simulink model "currloop"  (R2021b)
settings: Solver=FixedStepAuto  StartTime=0.0  StopTime=10.0  FixedStep=1e-4  RelTol=1e-3
undefined symbols (not defined in the file or in its folder): CurrKi, CurrKp, DiscIntNeverNeededParam, Pn, Ubus
libraries: slpidlib x4, mcbplantlib x1, autolibpmsmexterior x1
settings Model: DataDictionary=currloop.sldd  Creator=ssc  LastModifiedBy=ssc
settings OptimizationCC: DefaultParameterBehavior=Inlined  UseDivisionForNetSlopeComputation=on  GainParamInheritBuiltInType=on  UseFloatMulNetSlope=on  InlineInvariantSignals=on  PassReuseOutputArgsAs=Individual arguments  ZeroExternalMemoryAtStartup=off  ZeroInternalMemoryAtStartup=off  NoFixptDivByZeroProtection=on  EfficientFloat2IntCast=on  LifeSpan=1  OptimizeBlockOrder=speed  DifferentSizesBufferReuse=on  EfficientTunableParamExpr=on
settings DebuggingCC: ParameterTunabilityLossMsg=error
settings HardwareCC: ProdBitPerPointer=32  ProdBitPerSizeT=32  ProdBitPerPtrDiffT=32  ProdLargestAtomicInteger=Long  ProdLargestAtomicFloat=Double  ProdWordSize=32  ProdLongLongMode=on  ProdHWDeviceType=ARM Compatible->ARM Cortex-M
settings SFSimCC: MATLABDynamicMemAlloc=off
settings RTWCC: Description=Embedded Coder  SystemTargetFile=ert.tlc  TemplateMakefile=ert_default_tmf  GenerateReport=on  LaunchReport=on
settings CodeAppCC: ForceParamTrailComments=on  IgnoreCustomStorageClasses=off  OperatorAnnotations=on  SimulinkDataObjDesc=on  SFDataObjDesc=on  CustomSymbolStrGlobalVar=rt$N$M  CustomSymbolStrType=$N$M  CustomSymbolStrFcn=$N$M$F  CustomSymbolStrMacro=$N$M  InsertBlockDesc=on
settings ERTTargetCC: TargetLangStandard=C99 (ISO)  CodeReplacementLibrary=ARM Cortex-M  GenerateSampleERTMain=on  IncludeMdlTerminateFcn=off  CombineSignalStateStructs=on  SupportAbsoluteTime=off  SupportComplex=off  SupportContinuousTime=on  SupportNonInlinedSFcns=on  InlinedParameterPlacement=NonHierarchical  ERTCustomFileTemplate=example_file_process.tlc  ERTFilePackagingFormat=CompactWithDataFile

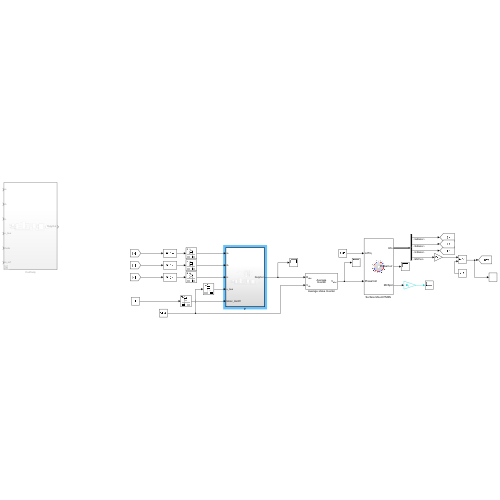
[thumbnail: Simulink's stored preview of the top-level diagram]
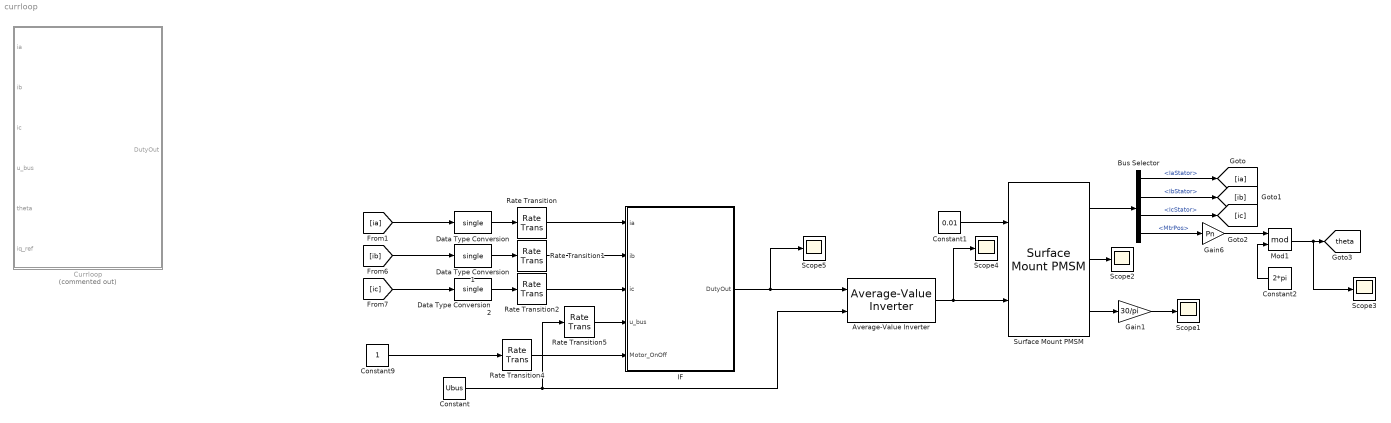
== system currloop ==
  Average-Value Inverter : mcbplantlib/Average-Value Inverter
  Bus Selector : BusSelector  OutputSignals=IaStator,IbStator,IcStator,MtrPos
  Constant : Constant  Value=Ubus
  Constant1 : Constant  Value=0.01
  Constant2 : Constant  Value=2*pi  OutDataTypeStr=single
  Constant9 : Constant
  Currloop : Subsystem  Commented=on  TreatAsAtomicUnit=on
  Data Type Conversion : DataTypeConversion  OutDataTypeStr=single
  Data Type Conversion1 : DataTypeConversion  OutDataTypeStr=single
  Data Type Conversion2 : DataTypeConversion  OutDataTypeStr=single
  Gain1 : Gain  Gain=30/pi  OutDataTypeStr=single
  Gain6 : Gain  Gain=Pn  OutDataTypeStr=single
  IF : Subsystem  TreatAsAtomicUnit=on
  Mod1 : Math  Operator=mod  OutputSignalType=real  SaturateOnIntegerOverflow=on
  Rate Transition{,1..2,4..5} (5 alike) : RateTransition
  Scope{1..5} (5 alike) : Scope
  Surface Mount PMSM : autolibpmsmexterior/Surface Mount PMSM  port_config=Torque  sim_type=Continuous  Ts=0.001  P=Pn  Rs=Rs  Ldq_=L  KConstText=Permanent flux linkage constant (lambda_pm):  lambda_pm=flux  Ke=159.9771  Kt=1.323  mechanical=[75e-6,8e-5,0]  idq0=[0 0]  theta_init=0  omega_init=0  KConst=flux  lambda_pm_calc=flux  RefBlkName='autolibpmsmexterior/Surface Mount PMSM'  aMode=5  Ldq="[0.0017      0.0017]"
      settings: SourceProductBaseCode=PW,DR,MT,UV,VE
  tag scope: theta=global
  wires:
  Average-Value Inverter/1 -> Scope4/1, Surface Mount PMSM/2
  Constant/1 -> Average-Value Inverter/2, Rate Transition5/1
  Mod1/1 -> Scope3/1, [theta]
  Bus Selector/1 -> [ia]  "<IaStator>"
  Bus Selector/4 -> Gain6/1  "<MtrPos>"
  Constant2/1 -> Mod1/2
  Surface Mount PMSM/1 -> Bus Selector/1
  Gain6/1 -> Mod1/1
  Bus Selector/3 -> [ic]  "<IcStator>"
  Bus Selector/2 -> [ib]  "<IbStator>"
  Data Type Conversion1/1 -> Rate Transition1/1
  Data Type Conversion/1 -> Rate Transition/1
  [ic] -> Data Type Conversion2/1
  [ia] -> Data Type Conversion/1
  [ib] -> Data Type Conversion1/1
  Data Type Conversion2/1 -> Rate Transition2/1
  Surface Mount PMSM/3 -> Gain1/1
  Gain1/1 -> Scope1/1
  Surface Mount PMSM/2 -> Scope2/1
  Constant9/1 -> Rate Transition4/1
  Rate Transition5/1 -> IF/4(u_bus)
  Rate Transition4/1 -> IF/5(Motor_OnOff)
  Rate Transition/1 -> IF/1(ia)
  Rate Transition1/1 -> IF/2(ib)
  Rate Transition2/1 -> IF/3(ic)
  IF/1(DutyOut) -> Scope5/1, Average-Value Inverter/1
  Constant1/1 -> Surface Mount PMSM/1

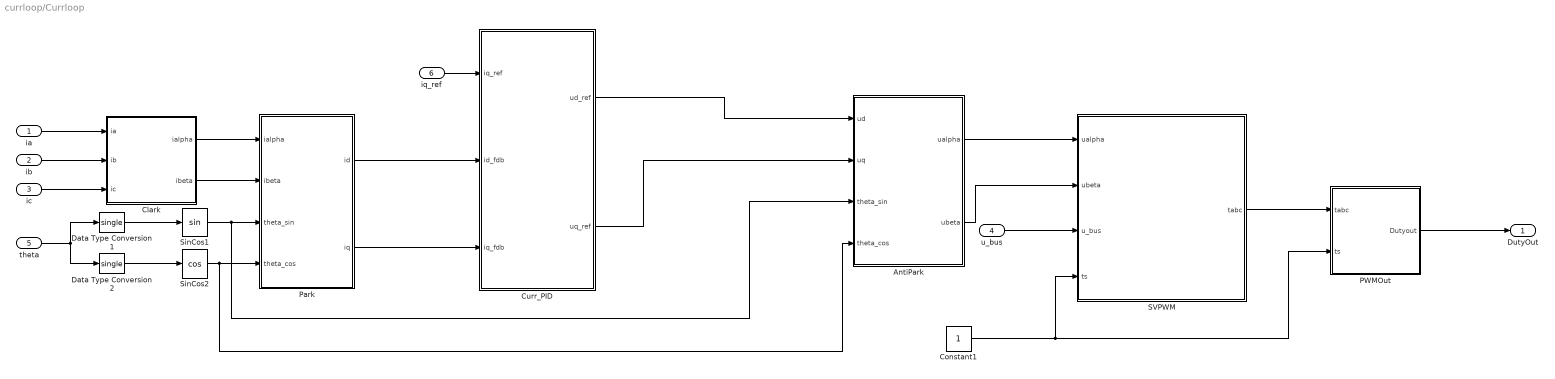
== system currloop/Currloop ==
  ia : Inport
  ib : Inport  Port=2
  ic : Inport  Port=3
  u_bus : Inport  Port=4
  theta : Inport  Port=5
  iq_ref : Inport  Port=6
  AntiPark : Subsystem
  Clark : Subsystem
  Constant1 : Constant
  Curr_PID : Subsystem
  Data Type Conversion1 : DataTypeConversion  OutDataTypeStr=single
  Data Type Conversion2 : DataTypeConversion  OutDataTypeStr=single
  PWMOut : Subsystem
  Park : Subsystem
  SVPWM : Subsystem
  SinCos1 : Trigonometry
  SinCos2 : Trigonometry  Operator=cos
  DutyOut : Outport
  wires:
  Constant1/1 -> PWMOut/2(ts), SVPWM/4(ts)
  SVPWM/1(tabc) -> PWMOut/1(tabc)
  u_bus/1 -> SVPWM/3(u_bus)
  PWMOut/1(Dutyout) -> DutyOut/1
  AntiPark/1(ualpha) -> SVPWM/1(ualpha)
  AntiPark/2(ubeta) -> SVPWM/2(ubeta)
  ia/1 -> Clark/1(ia)
  ib/1 -> Clark/2(ib)
  ic/1 -> Clark/3(ic)
  Clark/1(ialpha) -> Park/1(ialpha)
  Clark/2(ibeta) -> Park/2(ibeta)
  Park/1(id) -> Curr_PID/2(id_fdb)
  Park/2(iq) -> Curr_PID/3(iq_fdb)
  Data Type Conversion2/1 -> SinCos2/1
  Data Type Conversion1/1 -> SinCos1/1
  SinCos2/1 -> AntiPark/4(theta_cos), Park/4(theta_cos)
  SinCos1/1 -> AntiPark/3(theta_sin), Park/3(theta_sin)
  theta/1 -> Data Type Conversion1/1, Data Type Conversion2/1
  iq_ref/1 -> Curr_PID/1(iq_ref)
  Curr_PID/1(ud_ref) -> AntiPark/1(ud)
  Curr_PID/2(uq_ref) -> AntiPark/2(uq)

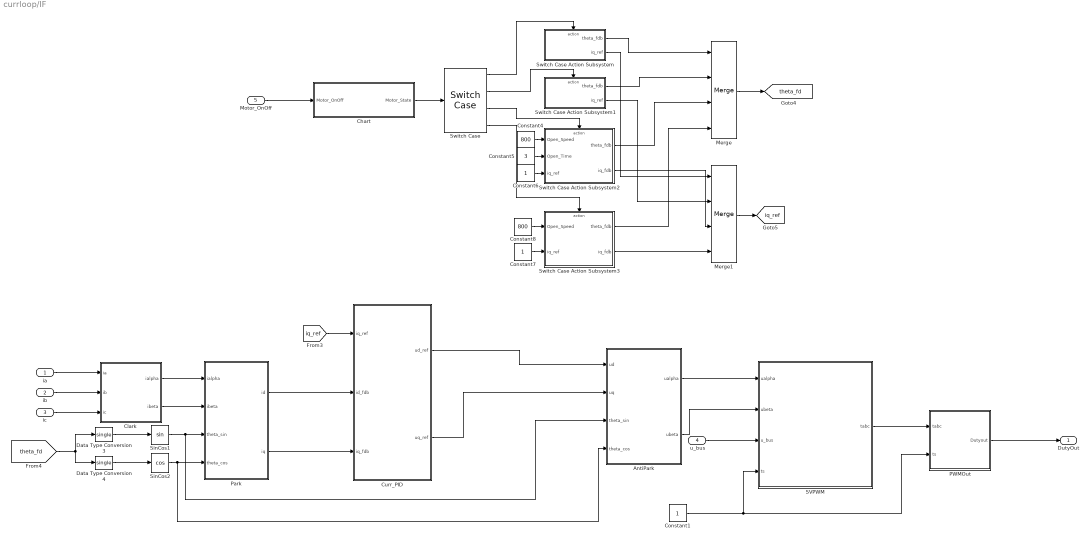
== system currloop/IF ==
  ia : Inport
  ib : Inport  Port=2
  ic : Inport  Port=3
  u_bus : Inport  Port=4
  Motor_OnOff : Inport  Port=5
  AntiPark : Subsystem
  Chart : Stateflow chart  TreatAsAtomicUnit=on
  Clark : Subsystem
  Constant1 : Constant
  Constant4 : Constant  Value=800
  Constant5 : Constant  Value=3
  Constant6 : Constant
  Constant7 : Constant
  Constant8 : Constant  Value=800
  Curr_PID : Subsystem
  Data Type Conversion3 : DataTypeConversion  OutDataTypeStr=single
  Data Type Conversion4 : DataTypeConversion  OutDataTypeStr=single
  Merge : Merge  Inputs=4
  Merge1 : Merge  Inputs=4
  PWMOut : Subsystem
  Park : Subsystem
  SVPWM : Subsystem
  SinCos1 : Trigonometry
  SinCos2 : Trigonometry  Operator=cos
  Switch Case : SwitchCase  CaseConditions={1,2,3,4}  ShowDefaultCase=off
  Switch Case Action Subsystem : Subsystem  TreatAsAtomicUnit=on
  Switch Case Action Subsystem1 : Subsystem  TreatAsAtomicUnit=on
  Switch Case Action Subsystem2 : Subsystem  TreatAsAtomicUnit=on
  Switch Case Action Subsystem3 : Subsystem  TreatAsAtomicUnit=on
  DutyOut : Outport
  tag scope: iq_ref=global, theta_fd=global
  wires:
  [iq_ref] -> Curr_PID/1(iq_ref)
  Switch Case/2 -> Switch Case Action Subsystem1/Action
  ib/1 -> Clark/2(ib)
  Park/1(id) -> Curr_PID/2(id_fdb)
  Curr_PID/1(ud_ref) -> AntiPark/1(ud)
  Clark/1(ialpha) -> Park/1(ialpha)
  Switch Case Action Subsystem/2(iq_ref) -> Merge1/1
  Data Type Conversion4/1 -> SinCos2/1
  Curr_PID/2(uq_ref) -> AntiPark/2(uq)
  [theta_fd] -> Data Type Conversion3/1, Data Type Conversion4/1
  SinCos2/1 -> AntiPark/4(theta_cos), Park/4(theta_cos)
  SinCos1/1 -> AntiPark/3(theta_sin), Park/3(theta_sin)
  AntiPark/1(ualpha) -> SVPWM/1(ualpha)
  ia/1 -> Clark/1(ia)
  Switch Case/4 -> Switch Case Action Subsystem3/Action
  Constant4/1 -> Switch Case Action Subsystem2/1(Open_Speed)
  Constant1/1 -> PWMOut/2(ts), SVPWM/4(ts)
  AntiPark/2(ubeta) -> SVPWM/2(ubeta)
  Constant8/1 -> Switch Case Action Subsystem3/1(Open_Speed)
  ic/1 -> Clark/3(ic)
  Clark/2(ibeta) -> Park/2(ibeta)
  Switch Case/3 -> Switch Case Action Subsystem2/Action
  Data Type Conversion3/1 -> SinCos1/1
  Switch Case Action Subsystem/1(theta_fdb) -> Merge/1
  SVPWM/1(tabc) -> PWMOut/1(tabc)
  Switch Case Action Subsystem1/1(theta_fdb) -> Merge/2
  Park/2(iq) -> Curr_PID/3(iq_fdb)
  u_bus/1 -> SVPWM/3(u_bus)
  Switch Case Action Subsystem3/1(theta_fdb) -> Merge/4
  Constant7/1 -> Switch Case Action Subsystem3/2(iq_ref)
  PWMOut/1(Dutyout) -> DutyOut/1
  Constant6/1 -> Switch Case Action Subsystem2/3(iq_ref)
  Switch Case/1 -> Switch Case Action Subsystem/Action
  Switch Case Action Subsystem3/2(iq_fdb) -> Merge1/4
  Merge1/1 -> [iq_ref]
  Constant5/1 -> Switch Case Action Subsystem2/2(Open_Time)
  Switch Case Action Subsystem1/2(iq_ref) -> Merge1/2
  Switch Case Action Subsystem2/1(theta_fdb) -> Merge/3
  Merge/1 -> [theta_fd]
  Switch Case Action Subsystem2/2(iq_fdb) -> Merge1/3
  Chart/1(Motor_State) -> Switch Case/1
  Motor_OnOff/1 -> Chart/1(Motor_OnOff)

== system currloop/Currloop/AntiPark ==
  ud : Inport
  uq : Inport  Port=2
  theta_sin : Inport  Port=3
  theta_cos : Inport  Port=4
  Product{,1..3} (4 alike) : Product
  Subtract : Sum
  Subtract1 : Sum  Inputs=-+
  ualpha : Outport
  ubeta : Outport  Port=2
  wires:
  ud/1 -> Product/1, Product3/1
  theta_sin/1 -> Product2/2, Product/2
  uq/1 -> Product1/1, Product2/1
  theta_cos/1 -> Product3/2, Product1/2
  Product/1 -> Subtract/1
  Product1/1 -> Subtract/2
  Product2/1 -> Subtract1/1
  Product3/1 -> Subtract1/2
  Subtract/1 -> ubeta/1
  Subtract1/1 -> ualpha/1

== system currloop/Currloop/Clark ==
  ia : Inport
  ib : Inport  Port=2
  ic : Inport  Port=3
  Add : Sum
  Add1 : Sum  Inputs=+-
  Add2 : Sum  Inputs=+-
  Gain : Gain  Gain=2/3
  Gain1 : Gain  Gain=1/3
  Gain2 : Gain  Gain=sqrt(3)/3
  ialpha : Outport
  ibeta : Outport  Port=2
  wires:
  ia/1 -> Gain/1
  ib/1 -> Add1/1, Add/1
  ic/1 -> Add1/2, Add/2
  Add/1 -> Gain1/1
  Add1/1 -> Gain2/1
  Gain1/1 -> Add2/2
  Gain/1 -> Add2/1
  Gain2/1 -> ibeta/1
  Add2/1 -> ialpha/1

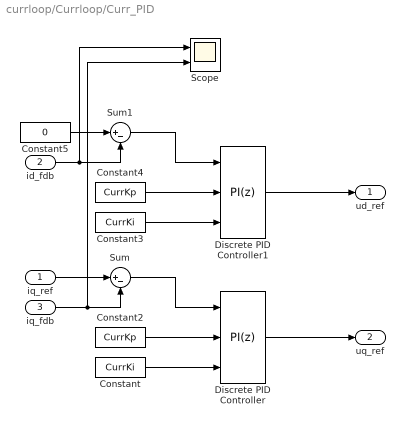
== system currloop/Currloop/Curr_PID ==
  iq_ref : Inport
  id_fdb : Inport  Port=2
  iq_fdb : Inport  Port=3
  Constant : Constant  Value=CurrKi
  Constant2 : Constant  Value=CurrKp
  Constant3 : Constant  Value=CurrKi
  Constant4 : Constant  Value=CurrKp
  Constant5 : Constant  Value=0
  Discrete PID Controller : slpidlib/PID Controller  Controller=PI  Form=Parallel  TimeDomain=Discrete-time  UseExternalTs=off  SampleTime=-1  IntegratorMethod=Forward Euler  FilterMethod=Forward Euler  ControllerParametersSource=external  P=1  I=1  D=0  UseFilter=on  N=100  TunerSelectOption=Transfer Function Based (PID Tuner App)  InitialConditionSource=internal  InitialConditionForIntegrator=0  InitialConditionForFilter=0  DifferentiatorICPrevScaledInput=0  ExternalReset=none  TrackingMode=off  Kt=1  LimitOutput=on  SatLimitsSource=internal  UpperSaturationLimit=Ubus/sqrt(3)  LowerSaturationLimit=-Ubus/sqrt(3)  LinearizeAsGain=off  AntiWindupMode=clamping  Kb=1  POutMin=[]  POutMax=[]  IOutMin=[]  IOutMax=[]  DOutMin=[]  DOutMax=[]  NOutMin=[]  NOutMax=[]  SumOutMin=[]  SumOutMax=[]  SaturationOutMin=[]  SaturationOutMax=[]  PParamMin=[]  PParamMax=[]  IParamMin=[]  IParamMax=[]  DParamMin=[]  DParamMax=[]  NParamMin=[]  NParamMax=[]  KbParamMin=[]  KbParamMax=[]  KtParamMin=[]  KtParamMax=[]  KbOutMin=[]  KbOutMax=[]  KtOutMin=[]  KtOutMax=[]  IntegratorOutMin=[]  IntegratorOutMax=[]  FilterOutMin=[]  FilterOutMax=[]  SumI1OutMin=[]  SumI1OutMax=[]  SumI2OutMin=[]  SumI2OutMax=[]  SumI3OutMin=[]  SumI3OutMax=[]  SumI4OutMin=[]  SumI4OutMax=[]  SumDOutMin=[]  SumDOutMax=[]  DifferentiatorOutMin=[]  DifferentiatorOutMax=[]  FilterDiffOutCoefMin=[]  FilterDiffOutCoefMax=[]  ReciprocalOutMin=[]  ReciprocalOutMax=[]  SumDenOutMin=[]  SumDenOutMax=[]  SumNumOutMin=[]  SumNumOutMax=[]  DivideOutMin=[]  DivideOutMax=[]  UdiffTsProdOutMin=[]  UdiffTsProdOutMax=[]  NTsProdOutMin=[]  NTsProdOutMax=[]  UintegralTsProdOutMin=[]  UintegralTsProdOutMax=[]  UngainTsProdOutMin=[]  UngainTsProdOutMax=[]  IntegratorContinuousStateAttributes=''  IntegratorStateMustResolveToSignalObject=off  IntegratorRTWStateStorageClass=Auto  FilterContinuousStateAttributes=''  FilterStateMustResolveToSignalObject=off  FilterRTWStateStorageClass=Auto  ParallelPVariant=ExternalParameters  IdealPVariant=Disabled  IVariant=ExternalParameters  DVariant=Disabled  IntegratorVariant=Discrete  SatVariant=Enabled  AWVariant=DiscClampingParallel  PCopyVariant=Disabled  TRVariant=Disabled  FdbkBlocksVariant=Forward  IdealPFdbkVariant=Disabled  SatFdbkVariant=Disabled  DerivativeFilterVariant=Disabled  NVariant=Disabled  NCopyVariant=Disabled_SignalSpec  FilterICVariant=Disabled  IntegratorICVariant=InternalICs  ExternalResetVariant=Disabled  TRSumVariant=Passthrough  SumFdbkVariant=Disabled  SumVariant=Sum_PI  TsampFilterVariant=InternalTs  TsampNgainVariant=Passthrough  TsampIntegralVariant=Passthrough  ExternalSaturationOutDataTypeStr=Inherit: Same as second input
  Discrete PID Controller1 : slpidlib/PID Controller  Controller=PI  Form=Parallel  TimeDomain=Discrete-time  UseExternalTs=off  SampleTime=-1  IntegratorMethod=Forward Euler  FilterMethod=Forward Euler  ControllerParametersSource=external  P=1  I=1  D=0  UseFilter=on  N=100  TunerSelectOption=Transfer Function Based (PID Tuner App)  InitialConditionSource=internal  InitialConditionForIntegrator=0  InitialConditionForFilter=0  DifferentiatorICPrevScaledInput=0  ExternalReset=none  TrackingMode=off  Kt=1  LimitOutput=on  SatLimitsSource=internal  UpperSaturationLimit=Ubus/sqrt(3)  LowerSaturationLimit=-Ubus/sqrt(3)  LinearizeAsGain=off  AntiWindupMode=clamping  Kb=1  POutMin=[]  POutMax=[]  IOutMin=[]  IOutMax=[]  DOutMin=[]  DOutMax=[]  NOutMin=[]  NOutMax=[]  SumOutMin=[]  SumOutMax=[]  SaturationOutMin=[]  SaturationOutMax=[]  PParamMin=[]  PParamMax=[]  IParamMin=[]  IParamMax=[]  DParamMin=[]  DParamMax=[]  NParamMin=[]  NParamMax=[]  KbParamMin=[]  KbParamMax=[]  KtParamMin=[]  KtParamMax=[]  KbOutMin=[]  KbOutMax=[]  KtOutMin=[]  KtOutMax=[]  IntegratorOutMin=[]  IntegratorOutMax=[]  FilterOutMin=[]  FilterOutMax=[]  SumI1OutMin=[]  SumI1OutMax=[]  SumI2OutMin=[]  SumI2OutMax=[]  SumI3OutMin=[]  SumI3OutMax=[]  SumI4OutMin=[]  SumI4OutMax=[]  SumDOutMin=[]  SumDOutMax=[]  DifferentiatorOutMin=[]  DifferentiatorOutMax=[]  FilterDiffOutCoefMin=[]  FilterDiffOutCoefMax=[]  ReciprocalOutMin=[]  ReciprocalOutMax=[]  SumDenOutMin=[]  SumDenOutMax=[]  SumNumOutMin=[]  SumNumOutMax=[]  DivideOutMin=[]  DivideOutMax=[]  UdiffTsProdOutMin=[]  UdiffTsProdOutMax=[]  NTsProdOutMin=[]  NTsProdOutMax=[]  UintegralTsProdOutMin=[]  UintegralTsProdOutMax=[]  UngainTsProdOutMin=[]  UngainTsProdOutMax=[]  IntegratorContinuousStateAttributes=''  IntegratorStateMustResolveToSignalObject=off  IntegratorRTWStateStorageClass=Auto  FilterContinuousStateAttributes=''  FilterStateMustResolveToSignalObject=off  FilterRTWStateStorageClass=Auto  ParallelPVariant=ExternalParameters  IdealPVariant=Disabled  IVariant=ExternalParameters  DVariant=Disabled  IntegratorVariant=Discrete  SatVariant=Enabled  AWVariant=DiscClampingParallel  PCopyVariant=Disabled  TRVariant=Disabled  FdbkBlocksVariant=Forward  IdealPFdbkVariant=Disabled  SatFdbkVariant=Disabled  DerivativeFilterVariant=Disabled  NVariant=Disabled  NCopyVariant=Disabled_SignalSpec  FilterICVariant=Disabled  IntegratorICVariant=InternalICs  ExternalResetVariant=Disabled  TRSumVariant=Passthrough  SumFdbkVariant=Disabled  SumVariant=Sum_PI  TsampFilterVariant=InternalTs  TsampNgainVariant=Passthrough  TsampIntegralVariant=Passthrough  ExternalSaturationOutDataTypeStr=Inherit: Same as second input
  Scope : Scope  NumInputPorts=2
  Sum : Sum  Inputs=|+-
  Sum1 : Sum  Inputs=|+-
  ud_ref : Outport
  uq_ref : Outport  Port=2
  wires:
  Constant2/1 -> Discrete PID Controller/2
  Constant3/1 -> Discrete PID Controller1/3
  Sum1/1 -> Discrete PID Controller1/1
  Sum/1 -> Discrete PID Controller/1
  Constant/1 -> Discrete PID Controller/3
  iq_ref/1 -> Sum/1
  Discrete PID Controller/1 -> uq_ref/1
  Constant4/1 -> Discrete PID Controller1/2
  Discrete PID Controller1/1 -> ud_ref/1
  Constant5/1 -> Sum1/1
  iq_fdb/1 -> Scope/2, Sum/2
  id_fdb/1 -> Scope/1, Sum1/2

== system currloop/Currloop/PWMOut ==
  tabc : Inport
  ts : Inport  Port=2
  Add : Sum  Inputs=-+
  Add1 : Sum  Inputs=-+
  Add2 : Sum  Inputs=-+
  Demux : Demux  Outputs=3
  Divide : Product  Inputs=*/
  Divide1 : Product  Inputs=*/
  Divide2 : Product  Inputs=*/
  Gain : Gain  Gain=2
  Mux : Mux  Inputs=3
  Dutyout : Outport
  wires:
  tabc/1 -> Gain/1
  Gain/1 -> Demux/1
  ts/1 -> Add1/2, Add2/2, Add/2, Divide2/2, Divide1/2, Divide/2
  Demux/3 -> Add/1
  Add/1 -> Divide/1
  Divide/1 -> Mux/3  "Dutyc"
  Demux/1 -> Add2/1
  Add1/1 -> Divide1/1
  Add2/1 -> Divide2/1
  Demux/2 -> Add1/1
  Divide1/1 -> Mux/2  "Dutyb"
  Divide2/1 -> Mux/1  "Dutya"
  Mux/1 -> Dutyout/1

== system currloop/Currloop/Park ==
  ialpha : Inport
  ibeta : Inport  Port=2
  theta_sin : Inport  Port=3
  theta_cos : Inport  Port=4
  Product{,1..3} (4 alike) : Product
  Subtract : Sum
  Subtract1 : Sum  Inputs=-+
  id : Outport
  iq : Outport  Port=2
  wires:
  ialpha/1 -> Product2/1, Product/1
  theta_cos/1 -> Product/2, Product3/2
  ibeta/1 -> Product3/1, Product1/1
  theta_sin/1 -> Product1/2, Product2/2
  Product/1 -> Subtract/1
  Product1/1 -> Subtract/2
  Subtract/1 -> id/1
  Product2/1 -> Subtract1/1
  Product3/1 -> Subtract1/2
  Subtract1/1 -> iq/1

== system currloop/Currloop/SVPWM ==
  ualpha : Inport
  ubeta : Inport  Port=2
  u_bus : Inport  Port=3
  ts : Inport  Port=4
  N : Subsystem
  t4_t6 : Subsystem
  t_abc : Subsystem
  tabc : Outport
  wires:
  ubeta/1 -> t4_t6/2(ubeta), N/2(ubeta)
  t4_t6/1(t4) -> t_abc/1(t4)
  N/1(N) -> t_abc/4(N), t4_t6/4(N)
  ualpha/1 -> t4_t6/1(ualpha), N/1(ualpha)
  t4_t6/2(t6) -> t_abc/2(t6)
  u_bus/1 -> t4_t6/3(u_bus)
  ts/1 -> t_abc/3(ts), t4_t6/5(ts)
  t_abc/1(tabc) -> tabc/1

== system currloop/IF/AntiPark ==
  ud : Inport
  uq : Inport  Port=2
  theta_sin : Inport  Port=3
  theta_cos : Inport  Port=4
  Product{,1..3} (4 alike) : Product
  Subtract : Sum
  Subtract1 : Sum  Inputs=-+
  ualpha : Outport
  ubeta : Outport  Port=2
  wires:
  ud/1 -> Product/1, Product3/1
  theta_sin/1 -> Product2/2, Product/2
  uq/1 -> Product1/1, Product2/1
  theta_cos/1 -> Product3/2, Product1/2
  Product/1 -> Subtract/1
  Product1/1 -> Subtract/2
  Product2/1 -> Subtract1/1
  Product3/1 -> Subtract1/2
  Subtract/1 -> ubeta/1
  Subtract1/1 -> ualpha/1

== system currloop/IF/Clark ==
  ia : Inport
  ib : Inport  Port=2
  ic : Inport  Port=3
  Add : Sum
  Add1 : Sum  Inputs=+-
  Add2 : Sum  Inputs=+-
  Gain : Gain  Gain=2/3
  Gain1 : Gain  Gain=1/3
  Gain2 : Gain  Gain=sqrt(3)/3
  ialpha : Outport
  ibeta : Outport  Port=2
  wires:
  ia/1 -> Gain/1
  ib/1 -> Add1/1, Add/1
  ic/1 -> Add1/2, Add/2
  Add/1 -> Gain1/1
  Add1/1 -> Gain2/1
  Gain1/1 -> Add2/2
  Gain/1 -> Add2/1
  Gain2/1 -> ibeta/1
  Add2/1 -> ialpha/1

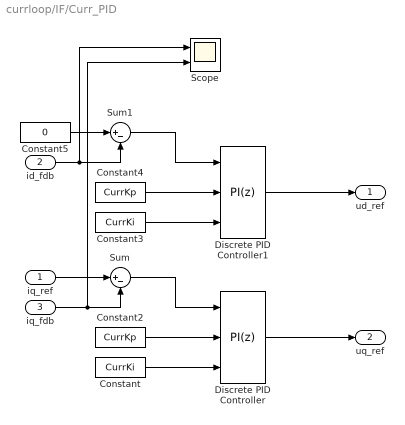
== system currloop/IF/Curr_PID ==
  iq_ref : Inport
  id_fdb : Inport  Port=2
  iq_fdb : Inport  Port=3
  Constant : Constant  Value=CurrKi
  Constant2 : Constant  Value=CurrKp
  Constant3 : Constant  Value=CurrKi
  Constant4 : Constant  Value=CurrKp
  Constant5 : Constant  Value=0
  Discrete PID Controller : slpidlib/PID Controller  Controller=PI  Form=Parallel  TimeDomain=Discrete-time  UseExternalTs=off  SampleTime=-1  IntegratorMethod=Forward Euler  FilterMethod=Forward Euler  ControllerParametersSource=external  P=1  I=1  D=0  UseFilter=on  N=100  TunerSelectOption=Transfer Function Based (PID Tuner App)  InitialConditionSource=internal  InitialConditionForIntegrator=0  InitialConditionForFilter=0  DifferentiatorICPrevScaledInput=0  ExternalReset=none  TrackingMode=off  Kt=1  LimitOutput=on  SatLimitsSource=internal  UpperSaturationLimit=Ubus/sqrt(3)  LowerSaturationLimit=-Ubus/sqrt(3)  LinearizeAsGain=off  AntiWindupMode=clamping  Kb=1  POutMin=[]  POutMax=[]  IOutMin=[]  IOutMax=[]  DOutMin=[]  DOutMax=[]  NOutMin=[]  NOutMax=[]  SumOutMin=[]  SumOutMax=[]  SaturationOutMin=[]  SaturationOutMax=[]  PParamMin=[]  PParamMax=[]  IParamMin=[]  IParamMax=[]  DParamMin=[]  DParamMax=[]  NParamMin=[]  NParamMax=[]  KbParamMin=[]  KbParamMax=[]  KtParamMin=[]  KtParamMax=[]  KbOutMin=[]  KbOutMax=[]  KtOutMin=[]  KtOutMax=[]  IntegratorOutMin=[]  IntegratorOutMax=[]  FilterOutMin=[]  FilterOutMax=[]  SumI1OutMin=[]  SumI1OutMax=[]  SumI2OutMin=[]  SumI2OutMax=[]  SumI3OutMin=[]  SumI3OutMax=[]  SumI4OutMin=[]  SumI4OutMax=[]  SumDOutMin=[]  SumDOutMax=[]  DifferentiatorOutMin=[]  DifferentiatorOutMax=[]  FilterDiffOutCoefMin=[]  FilterDiffOutCoefMax=[]  ReciprocalOutMin=[]  ReciprocalOutMax=[]  SumDenOutMin=[]  SumDenOutMax=[]  SumNumOutMin=[]  SumNumOutMax=[]  DivideOutMin=[]  DivideOutMax=[]  UdiffTsProdOutMin=[]  UdiffTsProdOutMax=[]  NTsProdOutMin=[]  NTsProdOutMax=[]  UintegralTsProdOutMin=[]  UintegralTsProdOutMax=[]  UngainTsProdOutMin=[]  UngainTsProdOutMax=[]  IntegratorContinuousStateAttributes=''  IntegratorStateMustResolveToSignalObject=off  IntegratorRTWStateStorageClass=Auto  FilterContinuousStateAttributes=''  FilterStateMustResolveToSignalObject=off  FilterRTWStateStorageClass=Auto  ParallelPVariant=ExternalParameters  IdealPVariant=Disabled  IVariant=ExternalParameters  DVariant=Disabled  IntegratorVariant=Discrete  SatVariant=Enabled  AWVariant=DiscClampingParallel  PCopyVariant=Disabled  TRVariant=Disabled  FdbkBlocksVariant=Forward  IdealPFdbkVariant=Disabled  SatFdbkVariant=Disabled  DerivativeFilterVariant=Disabled  NVariant=Disabled  NCopyVariant=Disabled_SignalSpec  FilterICVariant=Disabled  IntegratorICVariant=InternalICs  ExternalResetVariant=Disabled  TRSumVariant=Passthrough  SumFdbkVariant=Disabled  SumVariant=Sum_PI  TsampFilterVariant=InternalTs  TsampNgainVariant=Passthrough  TsampIntegralVariant=Passthrough  ExternalSaturationOutDataTypeStr=Inherit: Same as second input
  Discrete PID Controller1 : slpidlib/PID Controller  Controller=PI  Form=Parallel  TimeDomain=Discrete-time  UseExternalTs=off  SampleTime=-1  IntegratorMethod=Forward Euler  FilterMethod=Forward Euler  ControllerParametersSource=external  P=1  I=1  D=0  UseFilter=on  N=100  TunerSelectOption=Transfer Function Based (PID Tuner App)  InitialConditionSource=internal  InitialConditionForIntegrator=0  InitialConditionForFilter=0  DifferentiatorICPrevScaledInput=0  ExternalReset=none  TrackingMode=off  Kt=1  LimitOutput=on  SatLimitsSource=internal  UpperSaturationLimit=Ubus/sqrt(3)  LowerSaturationLimit=-Ubus/sqrt(3)  LinearizeAsGain=off  AntiWindupMode=clamping  Kb=1  POutMin=[]  POutMax=[]  IOutMin=[]  IOutMax=[]  DOutMin=[]  DOutMax=[]  NOutMin=[]  NOutMax=[]  SumOutMin=[]  SumOutMax=[]  SaturationOutMin=[]  SaturationOutMax=[]  PParamMin=[]  PParamMax=[]  IParamMin=[]  IParamMax=[]  DParamMin=[]  DParamMax=[]  NParamMin=[]  NParamMax=[]  KbParamMin=[]  KbParamMax=[]  KtParamMin=[]  KtParamMax=[]  KbOutMin=[]  KbOutMax=[]  KtOutMin=[]  KtOutMax=[]  IntegratorOutMin=[]  IntegratorOutMax=[]  FilterOutMin=[]  FilterOutMax=[]  SumI1OutMin=[]  SumI1OutMax=[]  SumI2OutMin=[]  SumI2OutMax=[]  SumI3OutMin=[]  SumI3OutMax=[]  SumI4OutMin=[]  SumI4OutMax=[]  SumDOutMin=[]  SumDOutMax=[]  DifferentiatorOutMin=[]  DifferentiatorOutMax=[]  FilterDiffOutCoefMin=[]  FilterDiffOutCoefMax=[]  ReciprocalOutMin=[]  ReciprocalOutMax=[]  SumDenOutMin=[]  SumDenOutMax=[]  SumNumOutMin=[]  SumNumOutMax=[]  DivideOutMin=[]  DivideOutMax=[]  UdiffTsProdOutMin=[]  UdiffTsProdOutMax=[]  NTsProdOutMin=[]  NTsProdOutMax=[]  UintegralTsProdOutMin=[]  UintegralTsProdOutMax=[]  UngainTsProdOutMin=[]  UngainTsProdOutMax=[]  IntegratorContinuousStateAttributes=''  IntegratorStateMustResolveToSignalObject=off  IntegratorRTWStateStorageClass=Auto  FilterContinuousStateAttributes=''  FilterStateMustResolveToSignalObject=off  FilterRTWStateStorageClass=Auto  ParallelPVariant=ExternalParameters  IdealPVariant=Disabled  IVariant=ExternalParameters  DVariant=Disabled  IntegratorVariant=Discrete  SatVariant=Enabled  AWVariant=DiscClampingParallel  PCopyVariant=Disabled  TRVariant=Disabled  FdbkBlocksVariant=Forward  IdealPFdbkVariant=Disabled  SatFdbkVariant=Disabled  DerivativeFilterVariant=Disabled  NVariant=Disabled  NCopyVariant=Disabled_SignalSpec  FilterICVariant=Disabled  IntegratorICVariant=InternalICs  ExternalResetVariant=Disabled  TRSumVariant=Passthrough  SumFdbkVariant=Disabled  SumVariant=Sum_PI  TsampFilterVariant=InternalTs  TsampNgainVariant=Passthrough  TsampIntegralVariant=Passthrough  ExternalSaturationOutDataTypeStr=Inherit: Same as second input
  Scope : Scope  NumInputPorts=2
  Sum : Sum  Inputs=|+-
  Sum1 : Sum  Inputs=|+-
  ud_ref : Outport
  uq_ref : Outport  Port=2
  wires:
  Constant2/1 -> Discrete PID Controller/2
  Constant3/1 -> Discrete PID Controller1/3
  Sum1/1 -> Discrete PID Controller1/1
  Sum/1 -> Discrete PID Controller/1
  Constant/1 -> Discrete PID Controller/3
  iq_ref/1 -> Sum/1
  Discrete PID Controller/1 -> uq_ref/1
  Constant4/1 -> Discrete PID Controller1/2
  Discrete PID Controller1/1 -> ud_ref/1
  Constant5/1 -> Sum1/1
  iq_fdb/1 -> Scope/2, Sum/2
  id_fdb/1 -> Scope/1, Sum1/2

== system currloop/IF/PWMOut ==
  tabc : Inport
  ts : Inport  Port=2
  Add : Sum  Inputs=-+
  Add1 : Sum  Inputs=-+
  Add2 : Sum  Inputs=-+
  Demux : Demux  Outputs=3
  Divide : Product  Inputs=*/
  Divide1 : Product  Inputs=*/
  Divide2 : Product  Inputs=*/
  Gain : Gain  Gain=2
  Mux : Mux  Inputs=3
  Dutyout : Outport
  wires:
  tabc/1 -> Gain/1
  Gain/1 -> Demux/1
  ts/1 -> Add1/2, Add2/2, Add/2, Divide2/2, Divide1/2, Divide/2
  Demux/3 -> Add/1
  Add/1 -> Divide/1
  Divide/1 -> Mux/3  "Dutyc"
  Demux/1 -> Add2/1
  Add1/1 -> Divide1/1
  Add2/1 -> Divide2/1
  Demux/2 -> Add1/1
  Divide1/1 -> Mux/2  "Dutyb"
  Divide2/1 -> Mux/1  "Dutya"
  Mux/1 -> Dutyout/1

== system currloop/IF/Park ==
  ialpha : Inport
  ibeta : Inport  Port=2
  theta_sin : Inport  Port=3
  theta_cos : Inport  Port=4
  Product{,1..3} (4 alike) : Product
  Subtract : Sum
  Subtract1 : Sum  Inputs=-+
  id : Outport
  iq : Outport  Port=2
  wires:
  ialpha/1 -> Product2/1, Product/1
  theta_cos/1 -> Product/2, Product3/2
  ibeta/1 -> Product3/1, Product1/1
  theta_sin/1 -> Product1/2, Product2/2
  Product/1 -> Subtract/1
  Product1/1 -> Subtract/2
  Subtract/1 -> id/1
  Product2/1 -> Subtract1/1
  Product3/1 -> Subtract1/2
  Subtract1/1 -> iq/1

== system currloop/IF/SVPWM ==
  ualpha : Inport
  ubeta : Inport  Port=2
  u_bus : Inport  Port=3
  ts : Inport  Port=4
  N : Subsystem
  t4_t6 : Subsystem
  t_abc : Subsystem
  tabc : Outport
  wires:
  ubeta/1 -> t4_t6/2(ubeta), N/2(ubeta)
  t4_t6/1(t4) -> t_abc/1(t4)
  N/1(N) -> t_abc/4(N), t4_t6/4(N)
  ualpha/1 -> t4_t6/1(ualpha), N/1(ualpha)
  t4_t6/2(t6) -> t_abc/2(t6)
  u_bus/1 -> t4_t6/3(u_bus)
  ts/1 -> t_abc/3(ts), t4_t6/5(ts)
  t_abc/1(tabc) -> tabc/1

== system currloop/IF/Switch Case Action Subsystem ==
  Action Port : ActionPort  ActionPortLabel=case [ 1 ]:
  Constant : Constant  Value=0
  Constant1 : Constant  Value=0
  theta_fdb : Outport
  iq_ref : Outport  Port=2
  wires:
  Constant/1 -> theta_fdb/1
  Constant1/1 -> iq_ref/1

== system currloop/IF/Switch Case Action Subsystem1 ==
  Action Port : ActionPort  ActionPortLabel=case [ 2 ]:
  Constant : Constant  Value=0
  Constant1 : Constant
  theta_fdb : Outport
  iq_ref : Outport  Port=2
  wires:
  Constant/1 -> theta_fdb/1
  Constant1/1 -> iq_ref/1

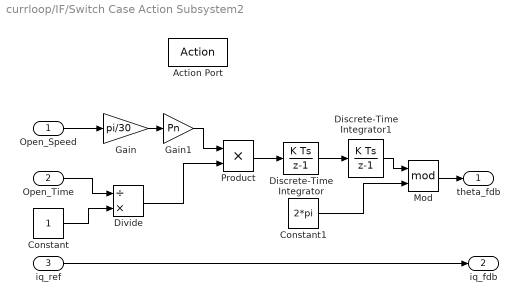
== system currloop/IF/Switch Case Action Subsystem2 ==
  Open_Speed : Inport
  Open_Time : Inport  Port=2
  iq_ref : Inport  Port=3
  Action Port : ActionPort  ActionPortLabel=case [ 3 ]:
  Constant : Constant
  Constant1 : Constant  Value=2*pi  OutDataTypeStr=double
  Discrete-Time Integrator : DiscreteIntegrator  SampleTime=-1  ICPrevOutput=DiscIntNeverNeededParam  ICPrevScaledInput=DiscIntNeverNeededParam
  Discrete-Time Integrator1 : DiscreteIntegrator  SampleTime=-1  ICPrevOutput=DiscIntNeverNeededParam  ICPrevScaledInput=DiscIntNeverNeededParam
  Divide : Product  Inputs=/*
  Gain : Gain  Gain=pi/30
  Gain1 : Gain  Gain=Pn
  Mod : Math  Operator=mod  SaturateOnIntegerOverflow=on
  Product : Product
  theta_fdb : Outport
  iq_fdb : Outport  Port=2
  wires:
  Open_Speed/1 -> Gain/1
  Gain/1 -> Gain1/1
  Gain1/1 -> Product/1
  Open_Time/1 -> Divide/1
  Constant/1 -> Divide/2
  Divide/1 -> Product/2
  Product/1 -> Discrete-Time Integrator/1
  iq_ref/1 -> iq_fdb/1
  Discrete-Time Integrator/1 -> Discrete-Time Integrator1/1
  Mod/1 -> theta_fdb/1
  Constant1/1 -> Mod/2
  Discrete-Time Integrator1/1 -> Mod/1

== system currloop/IF/Switch Case Action Subsystem3 ==
  Open_Speed : Inport
  iq_ref : Inport  Port=2
  Action Port : ActionPort  ActionPortLabel=case [ 4 ]:
  Constant1 : Constant  Value=2*pi  OutDataTypeStr=double
  Discrete-Time Integrator1 : DiscreteIntegrator  SampleTime=-1  ICPrevOutput=DiscIntNeverNeededParam  ICPrevScaledInput=DiscIntNeverNeededParam
  Gain : Gain  Gain=pi/30
  Gain1 : Gain  Gain=Pn
  Mod : Math  Operator=mod  SaturateOnIntegerOverflow=on
  theta_fdb : Outport
  iq_fdb : Outport  Port=2
  wires:
  Open_Speed/1 -> Gain/1
  Gain/1 -> Gain1/1
  iq_ref/1 -> iq_fdb/1
  Gain1/1 -> Discrete-Time Integrator1/1
  Constant1/1 -> Mod/2
  Discrete-Time Integrator1/1 -> Mod/1
  Mod/1 -> theta_fdb/1

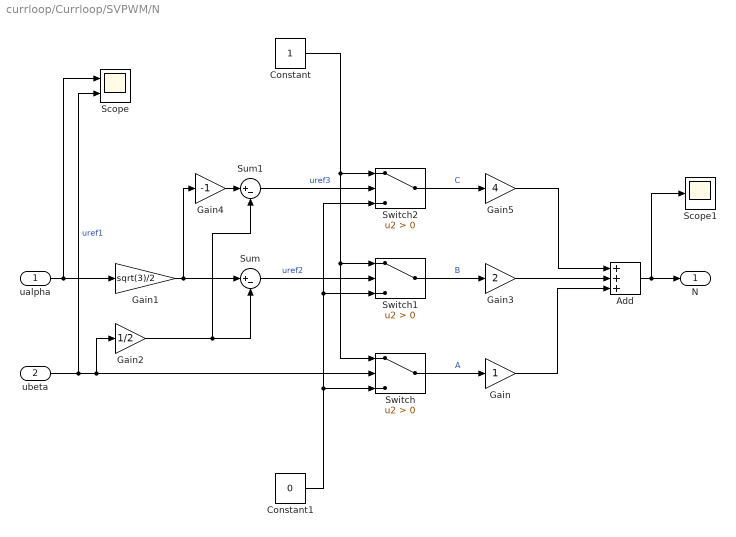
== system currloop/Currloop/SVPWM/N ==
  ualpha : Inport
  ubeta : Inport  Port=2
  Add : Sum  Inputs=+++
  Constant : Constant  OutDataTypeStr=single
  Constant1 : Constant  Value=0  OutDataTypeStr=single
  Gain : Gain
  Gain1 : Gain  Gain=sqrt(3)/2
  Gain2 : Gain  Gain=1/2
  Gain3 : Gain  Gain=2
  Gain4 : Gain  Gain=-1
  Gain5 : Gain  Gain=4
  Scope : Scope  NumInputPorts=2
  Scope1 : Scope
  Sum : Sum  Inputs=|+-
  Sum1 : Sum  Inputs=|+-
  Switch : Switch  Criteria=u2 > Threshold
  Switch1 : Switch  Criteria=u2 > Threshold
  Switch2 : Switch  Criteria=u2 > Threshold
  N : Outport
  wires:
  ualpha/1 -> Gain1/1, Scope/1
  ubeta/1 -> Switch/2, Gain2/1, Scope/2  "uref1"
  Constant/1 -> Switch2/1, Switch1/1, Switch/1
  Constant1/1 -> Switch2/3, Switch1/3, Switch/3
  Switch/1 -> Gain/1  "A"
  Gain1/1 -> Gain4/1, Sum/1
  Gain2/1 -> Sum1/2, Sum/2
  Sum/1 -> Switch1/2  "uref2"
  Switch1/1 -> Gain3/1  "B"
  Gain4/1 -> Sum1/1
  Sum1/1 -> Switch2/2  "uref3"
  Switch2/1 -> Gain5/1  "C"
  Gain3/1 -> Add/2
  Add/1 -> Scope1/1, N/1
  Gain/1 -> Add/3
  Gain5/1 -> Add/1

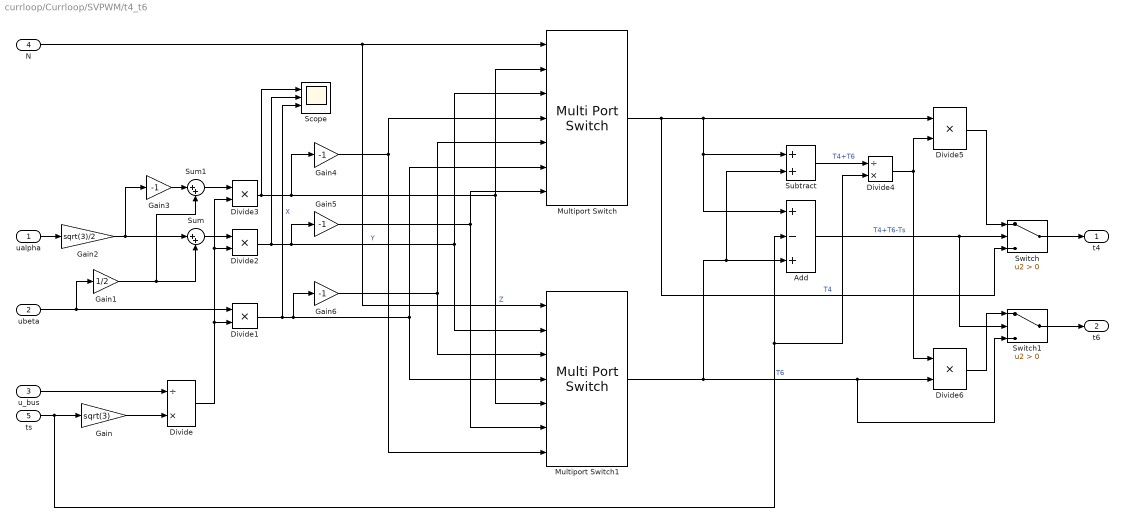
== system currloop/Currloop/SVPWM/t4_t6 ==
  ualpha : Inport
  ubeta : Inport  Port=2
  u_bus : Inport  Port=3
  N : Inport  Port=4
  ts : Inport  Port=5
  Add : Sum  Inputs=+-+
  Divide : Product  Inputs=/*
  Divide{1..3,5..6} (5 alike) : Product  Inputs=**
  Divide4 : Product  Inputs=/*
  Gain : Gain  Gain=sqrt(3)
  Gain1 : Gain  Gain=1/2
  Gain2 : Gain  Gain=sqrt(3)/2
  Gain{3..6} (4 alike) : Gain  Gain=-1
  Multiport Switch : MultiPortSwitch  Inputs=6
  Multiport Switch1 : MultiPortSwitch  Inputs=6
  Scope : Scope  NumInputPorts=3
  Subtract : Sum
  Sum : Sum  Inputs=|++
  Sum1 : Sum  Inputs=|++
  Switch : Switch  Criteria=u2 > Threshold
  Switch1 : Switch  Criteria=u2 > Threshold
  t4 : Outport
  t6 : Outport  Port=2
  wires:
  ts/1 -> Gain/1, Divide4/2, Add/2
  u_bus/1 -> Divide/1
  Gain/1 -> Divide/2
  ubeta/1 -> Gain1/1, Divide1/1
  Divide/1 -> Divide3/2, Divide2/2, Divide1/2
  Divide1/1 -> Scope/3, Multiport Switch1/4, Multiport Switch/6, Gain6/1  "X"
  ualpha/1 -> Gain2/1
  Gain1/1 -> Sum1/2, Sum/2
  Gain2/1 -> Gain3/1, Sum/1
  Sum/1 -> Divide2/1
  Divide2/1 -> Scope/2, Multiport Switch1/2, Multiport Switch/3, Gain5/1  "Y"
  Gain3/1 -> Sum1/1
  Sum1/1 -> Divide3/1
  Divide3/1 -> Scope/1, Gain4/1, Multiport Switch1/5, Multiport Switch/2  "Z"
  N/1 -> Multiport Switch1/1, Multiport Switch/1
  Multiport Switch/1 -> Switch/3, Divide5/1, Subtract/1, Add/1  "T4"
  Gain6/1 -> Multiport Switch1/3, Multiport Switch/5
  Gain4/1 -> Multiport Switch1/7, Multiport Switch/4
  Gain5/1 -> Multiport Switch1/6, Multiport Switch/7
  Add/1 -> Switch1/2, Switch/2  "T4+T6-Ts"
  Multiport Switch1/1 -> Switch1/3, Divide6/2, Subtract/2, Add/3  "T6"
  Subtract/1 -> Divide4/1  "T4+T6"
  Divide4/1 -> Divide5/2, Divide6/1
  Divide5/1 -> Switch/1
  Divide6/1 -> Switch1/1
  Switch/1 -> t4/1
  Switch1/1 -> t6/1

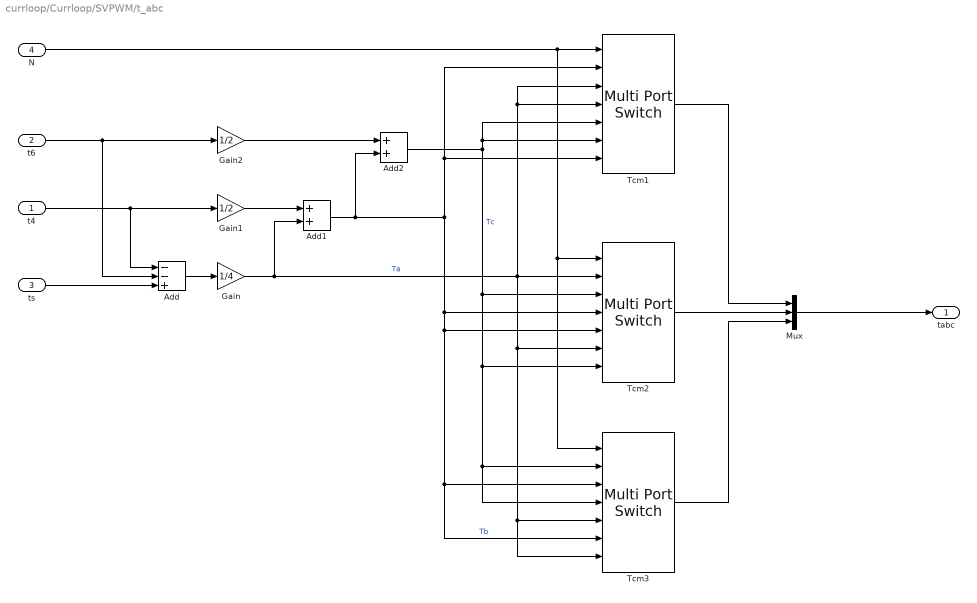
== system currloop/Currloop/SVPWM/t_abc ==
  t4 : Inport
  t6 : Inport  Port=2
  ts : Inport  Port=3
  N : Inport  Port=4
  Add : Sum  Inputs=--+
  Add1 : Sum
  Add2 : Sum
  Gain : Gain  Gain=1/4
  Gain1 : Gain  Gain=1/2
  Gain2 : Gain  Gain=1/2
  Mux : Mux  Inputs=3
  "Tcm1 " : MultiPortSwitch  Inputs=6
  Tcm2 : MultiPortSwitch  Inputs=6
  Tcm3 : MultiPortSwitch  Inputs=6
  tabc : Outport
  wires:
  ts/1 -> Add/3
  t6/1 -> Add/2, Gain2/1
  t4/1 -> Add/1, Gain1/1
  Add/1 -> Gain/1
  Gain/1 -> Tcm2/6, Tcm3/7, Tcm3/5, "Tcm1 "/4, "Tcm1 "/3, Tcm2/2, Add1/2  "Ta"
  Gain1/1 -> Add1/1
  Gain2/1 -> Add2/1
  Add1/1 -> Add2/2, "Tcm1 "/7, "Tcm1 "/2, Tcm2/4, Tcm3/6, Tcm3/3, Tcm2/5  "Tb"
  N/1 -> Tcm3/1, Tcm2/1, "Tcm1 "/1
  Add2/1 -> "Tcm1 "/6, "Tcm1 "/5, Tcm3/4, Tcm3/2, Tcm2/7, Tcm2/3  "Tc"
  "Tcm1 "/1 -> Mux/1
  Tcm3/1 -> Mux/3
  Tcm2/1 -> Mux/2
  Mux/1 -> tabc/1

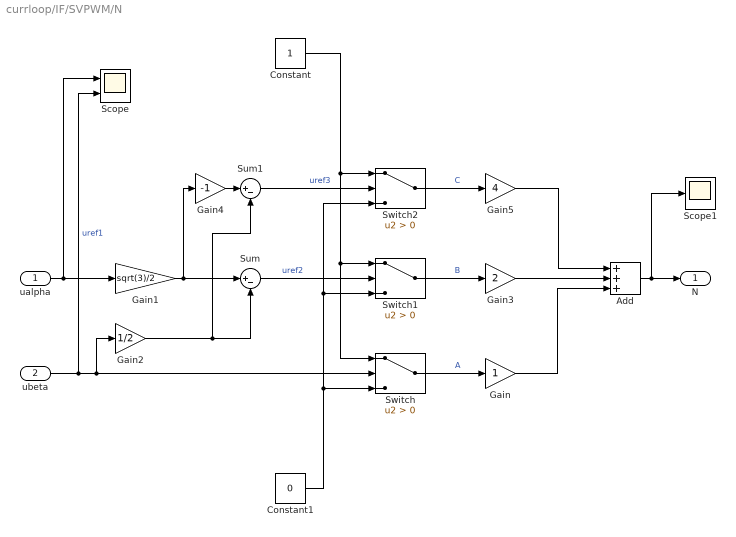
== system currloop/IF/SVPWM/N ==
  ualpha : Inport
  ubeta : Inport  Port=2
  Add : Sum  Inputs=+++
  Constant : Constant  OutDataTypeStr=single
  Constant1 : Constant  Value=0  OutDataTypeStr=single
  Gain : Gain
  Gain1 : Gain  Gain=sqrt(3)/2
  Gain2 : Gain  Gain=1/2
  Gain3 : Gain  Gain=2
  Gain4 : Gain  Gain=-1
  Gain5 : Gain  Gain=4
  Scope : Scope  NumInputPorts=2
  Scope1 : Scope
  Sum : Sum  Inputs=|+-
  Sum1 : Sum  Inputs=|+-
  Switch : Switch  Criteria=u2 > Threshold
  Switch1 : Switch  Criteria=u2 > Threshold
  Switch2 : Switch  Criteria=u2 > Threshold
  N : Outport
  wires:
  ualpha/1 -> Gain1/1, Scope/1
  ubeta/1 -> Switch/2, Gain2/1, Scope/2  "uref1"
  Constant/1 -> Switch2/1, Switch1/1, Switch/1
  Constant1/1 -> Switch2/3, Switch1/3, Switch/3
  Switch/1 -> Gain/1  "A"
  Gain1/1 -> Gain4/1, Sum/1
  Gain2/1 -> Sum1/2, Sum/2
  Sum/1 -> Switch1/2  "uref2"
  Switch1/1 -> Gain3/1  "B"
  Gain4/1 -> Sum1/1
  Sum1/1 -> Switch2/2  "uref3"
  Switch2/1 -> Gain5/1  "C"
  Gain3/1 -> Add/2
  Add/1 -> Scope1/1, N/1
  Gain/1 -> Add/3
  Gain5/1 -> Add/1

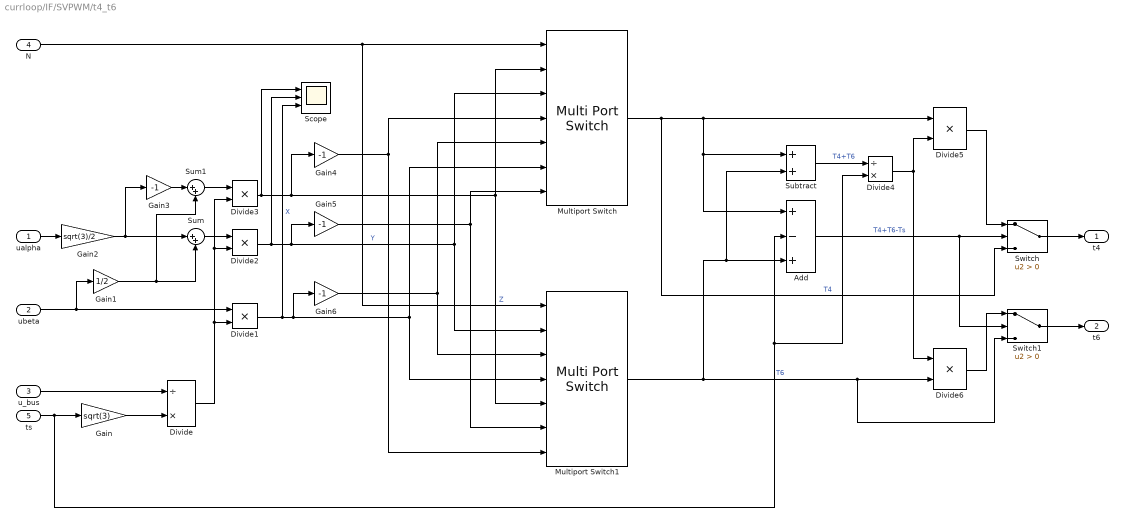
== system currloop/IF/SVPWM/t4_t6 ==
  ualpha : Inport
  ubeta : Inport  Port=2
  u_bus : Inport  Port=3
  N : Inport  Port=4
  ts : Inport  Port=5
  Add : Sum  Inputs=+-+
  Divide : Product  Inputs=/*
  Divide{1..3,5..6} (5 alike) : Product  Inputs=**
  Divide4 : Product  Inputs=/*
  Gain : Gain  Gain=sqrt(3)
  Gain1 : Gain  Gain=1/2
  Gain2 : Gain  Gain=sqrt(3)/2
  Gain{3..6} (4 alike) : Gain  Gain=-1
  Multiport Switch : MultiPortSwitch  Inputs=6  DiagnosticForDefault=None
  Multiport Switch1 : MultiPortSwitch  Inputs=6  DiagnosticForDefault=None
  Scope : Scope  NumInputPorts=3
  Subtract : Sum
  Sum : Sum  Inputs=|++
  Sum1 : Sum  Inputs=|++
  Switch : Switch  Criteria=u2 > Threshold
  Switch1 : Switch  Criteria=u2 > Threshold
  t4 : Outport
  t6 : Outport  Port=2
  wires:
  ts/1 -> Gain/1, Divide4/2, Add/2
  u_bus/1 -> Divide/1
  Gain/1 -> Divide/2
  ubeta/1 -> Gain1/1, Divide1/1
  Divide/1 -> Divide3/2, Divide2/2, Divide1/2
  Divide1/1 -> Scope/3, Multiport Switch1/4, Multiport Switch/6, Gain6/1  "X"
  ualpha/1 -> Gain2/1
  Gain1/1 -> Sum1/2, Sum/2
  Gain2/1 -> Gain3/1, Sum/1
  Sum/1 -> Divide2/1
  Divide2/1 -> Scope/2, Multiport Switch1/2, Multiport Switch/3, Gain5/1  "Y"
  Gain3/1 -> Sum1/1
  Sum1/1 -> Divide3/1
  Divide3/1 -> Scope/1, Gain4/1, Multiport Switch1/5, Multiport Switch/2  "Z"
  N/1 -> Multiport Switch1/1, Multiport Switch/1
  Multiport Switch/1 -> Switch/3, Divide5/1, Subtract/1, Add/1  "T4"
  Gain6/1 -> Multiport Switch1/3, Multiport Switch/5
  Gain4/1 -> Multiport Switch1/7, Multiport Switch/4
  Gain5/1 -> Multiport Switch1/6, Multiport Switch/7
  Add/1 -> Switch1/2, Switch/2  "T4+T6-Ts"
  Multiport Switch1/1 -> Switch1/3, Divide6/2, Subtract/2, Add/3  "T6"
  Subtract/1 -> Divide4/1  "T4+T6"
  Divide4/1 -> Divide5/2, Divide6/1
  Divide5/1 -> Switch/1
  Divide6/1 -> Switch1/1
  Switch/1 -> t4/1
  Switch1/1 -> t6/1

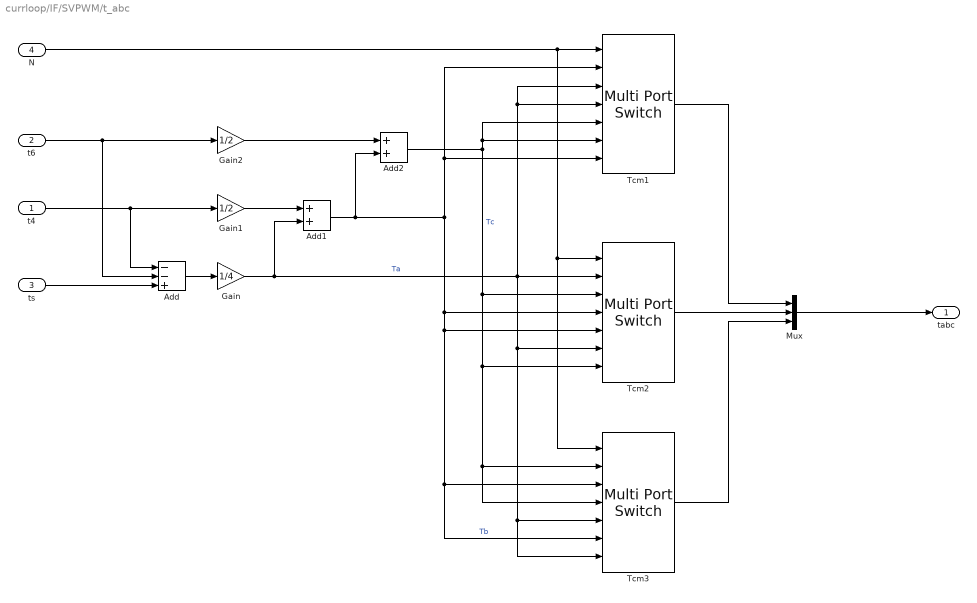
== system currloop/IF/SVPWM/t_abc ==
  t4 : Inport
  t6 : Inport  Port=2
  ts : Inport  Port=3
  N : Inport  Port=4
  Add : Sum  Inputs=--+
  Add1 : Sum
  Add2 : Sum
  Gain : Gain  Gain=1/4
  Gain1 : Gain  Gain=1/2
  Gain2 : Gain  Gain=1/2
  Mux : Mux  Inputs=3
  "Tcm1 " : MultiPortSwitch  Inputs=6  DiagnosticForDefault=None
  Tcm2 : MultiPortSwitch  Inputs=6  DiagnosticForDefault=None
  Tcm3 : MultiPortSwitch  Inputs=6  DiagnosticForDefault=None
  tabc : Outport
  wires:
  ts/1 -> Add/3
  t6/1 -> Add/2, Gain2/1
  t4/1 -> Add/1, Gain1/1
  Add/1 -> Gain/1
  Gain/1 -> Tcm2/6, Tcm3/7, Tcm3/5, "Tcm1 "/4, "Tcm1 "/3, Tcm2/2, Add1/2  "Ta"
  Gain1/1 -> Add1/1
  Gain2/1 -> Add2/1
  Add1/1 -> Add2/2, "Tcm1 "/7, "Tcm1 "/2, Tcm2/4, Tcm3/6, Tcm3/3, Tcm2/5  "Tb"
  N/1 -> Tcm3/1, Tcm2/1, "Tcm1 "/1
  Add2/1 -> "Tcm1 "/6, "Tcm1 "/5, Tcm3/4, Tcm3/2, Tcm2/7, Tcm2/3  "Tc"
  "Tcm1 "/1 -> Mux/1
  Tcm3/1 -> Mux/3
  Tcm2/1 -> Mux/2
  Mux/1 -> tabc/1

== stateflow chart currloop/IF/Chart ==
  state IDLE
    en:
    du:
    Motor_State = 1;
  state RunStage
    en:
    du:
    Motor_State = 4;
  state AlignStage
    en:
    du:
    Motor_State = 2;
  state OpenStage
    en:
    du:
    Motor_State = 3;
  (default) -> IDLE
  OpenStage -> RunStage [order 1] : [after(30000,tick)]
  IDLE -> AlignStage : [Motor_OnOff == 1]
  AlignStage -> OpenStage [order 1] : [after(1000,tick)]
  RunStage -> IDLE : [Motor_OnOff == 0]
  AlignStage -> IDLE [order 2] : [Motor_OnOff == 0]
  OpenStage -> IDLE [order 2] : [Motor_OnOff == 0]
  data: Motor_OnOff input; Motor_State output
